simulink model "uprugost"  (R2021b)
settings: Solver=FixedStepAuto  StartTime=0.0  StopTime=30.0  RelTol=1e-3
libraries: commrandsrc3 x1, commdigbbndam3 x1
settings Model: Creator=ksksks  LastModifiedBy=ksksks

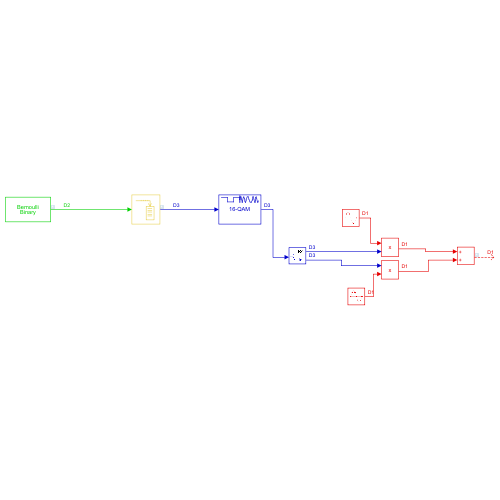
[thumbnail: Simulink's stored preview of the top-level diagram]
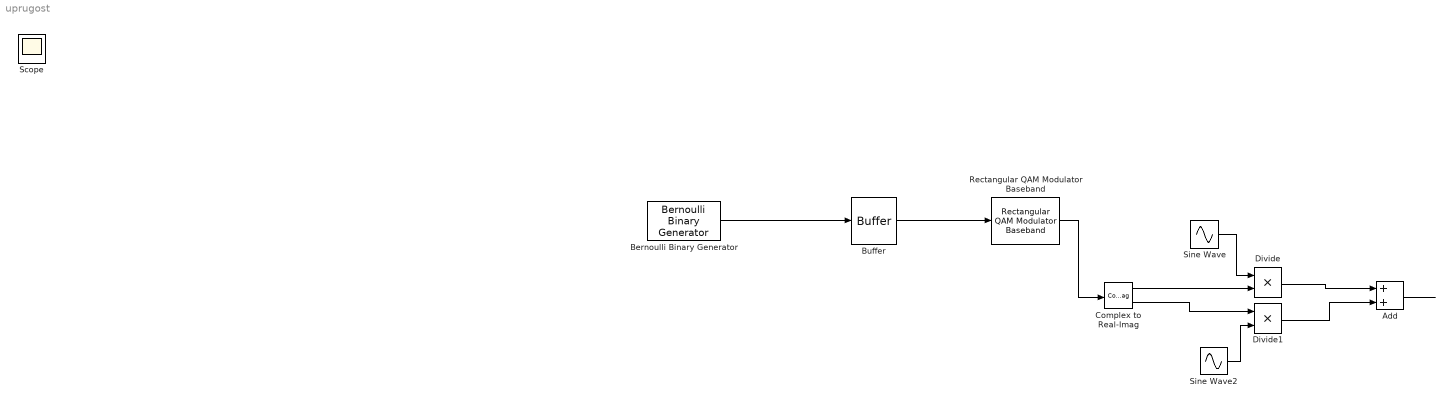
== system uprugost ==
  Add : Sum
  Bernoulli Binary Generator : commrandsrc3/Bernoulli Binary Generator  ProbabilityOfZero=0.5  SeedSource=Auto  Seed=0  SampleTime=1e-6  SamplesPerFrame=1  OutputDataType=double  SimulateUsing=Interpreted execution
  Buffer : Buffer  N=4  OutputFrames=off
  Complex to Real-Imag : ComplexToRealImag
  Divide : Product  Inputs=**
  Divide1 : Product  Inputs=**
  Rectangular QAM Modulator Baseband : commdigbbndam3/Rectangular QAM Modulator Baseband  M=16  InType=Bit  Enc=Gray  Mapping=[0:15]  PowType=Min. distance between symbols  MinDist=2  AvgPow=1  PeakPow=1  Ph=0  outDtype=double  outWordLen=16  outUDDataType=sfix(16)  outFracLenMode=Best precision  outFracLen=15  outDataTypeStr=double  outLastDataTypeStr=double
  Sine Wave : Sin  SineType=Sample based  Samples=20  SampleTime=1e-8
  Sine Wave2 : Sin  SineType=Sample based  Samples=20  SampleTime=1e-8  Offset=5
  Scope : Scope
  wires:
  Bernoulli Binary Generator/1 -> Buffer/1
  Buffer/1 -> Rectangular QAM Modulator Baseband/1
  Rectangular QAM Modulator Baseband/1 -> Complex to Real-Imag/1
  Complex to Real-Imag/1 -> Divide/2
  Sine Wave/1 -> Divide/1
  Complex to Real-Imag/2 -> Divide1/1
  Sine Wave2/1 -> Divide1/2
  Divide/1 -> Add/1
  Divide1/1 -> Add/2
  Add/1 -> ?
